simulink model "SingleTrack"  (R2019b)
settings: Solver=ode1  StartTime=0  StopTime=250  FixedStep=1.0000000000000000e-003  RelTol=1e-3
InitFcn:
  | sampleTime = str2double(get_param(bdroot, 'FixedStep'));
undefined symbols (not defined in the file or in its folder): AccPedalPos, BrakePedalPos, BrakeSwitch, DiscIntNeverNeededParam, DYNA4, EngSpd, IgnitionSwitch, InitialGear, InitialSpeed, IntendedEngTrq, LeftIndicator, MainBrakePress, MaxGear, MDL, MinGear, RefAcc, RefLane, RefLatPos, RefPath, RefPathCurv, RefSpd, RefSpdPreview, RefSpdRetrospect, RightIndicator, SteeringWheelAng, SteeringWheelTrq, UserDefinedRefValue, vm_const
libraries: UtilitiesLibrary x31, simulink x18, WheelSystemModules x13, LongitudinalControllerModules x13, LateralControllerModules x7, AnimationBusselectorModules x5, EnvironmentModules x5, BasicEngineControlModules x5, MiscellaneousControlModules x5, Animation3Modules x4, AuxiliariesModules x4, ReducedTireModules x4
(part 32 of 32)

== system SingleTrack/VehicleControl/LongitudinalControl/ControlSystems/Longitudinal Controller/Speed Control/Load Torque Vehicle ==
  VehSpd[m/s] : Inport
  TireRadius[m] : Inport  Port=2
  AerodynamicFrc[N] : Inport  Description=Vehicle Velocity  Port=3
  RoadSlopeLong [-] : Inport  Port=4
  SumMaxRollResistanceTrq[Nm] : Inport  Description=Vehicle Velocity  Port=5
  VehMass [kg] : Inport  Port=6
  BrakeFrc[N] : Inport  Port=7
  Constant : Constant  Value=9.81
  F_load [N] : Sum  Inputs=3  SaturateOnIntegerOverflow=on  InputSameDT=on  OutDataTypeStr=Inherit: Same as first input
  LoadTrq : Product  SaturateOnIntegerOverflow=on  InputSameDT=on  OutDataTypeStr=Inherit: Same as first input
  Resist.Torque : Product  SaturateOnIntegerOverflow=on  InputSameDT=on  OutDataTypeStr=Inherit: Same as first input
  Slope Force : Product  Inputs=3  SaturateOnIntegerOverflow=on  InputSameDT=on  OutDataTypeStr=Inherit: Same as first input
  Trigonometric Function : Trigonometry
  Trigonometric Function1 : Trigonometry  Operator=atan
  abs(F_load) [N]1 : Sum  Inputs=2  SaturateOnIntegerOverflow=on  InputSameDT=on  OutDataTypeStr=Inherit: Same as first input
  fade out load torque if speed is zero : Saturate  UpperLimit=1  LowerLimit=0
  toCompile : Subsystem  Tag=em_compile_service
      settings: AttributesFormatString=Place this block in the subsystem\n you want to compile
  LoadTrq[Nm] : Outport  VectorParamsAs1DForOutWhenUnconnected=off
  wires:
  VehSpd[m/s]/1 -> fade out load torque if speed is zero/1
  SumMaxRollResistanceTrq[Nm]/1 -> abs(F_load) [N]1/2
  TireRadius[m]/1 -> Resist.Torque/2
  Slope Force/1 -> F_load [N]/3
  Trigonometric Function/1 -> Slope Force/3
  VehMass [kg]/1 -> Slope Force/2
  Constant/1 -> Slope Force/1
  AerodynamicFrc[N]/1 -> F_load [N]/1
  BrakeFrc[N]/1 -> F_load [N]/2
  Resist.Torque/1 -> abs(F_load) [N]1/1
  RoadSlopeLong [-]/1 -> Trigonometric Function1/1
  F_load [N]/1 -> Resist.Torque/1
  abs(F_load) [N]1/1 -> LoadTrq/2
  fade out load torque if speed is zero/1 -> LoadTrq/1
  LoadTrq/1 -> LoadTrq[Nm]/1
  Trigonometric Function1/1 -> Trigonometric Function/1

== system SingleTrack/VehicleControl/LongitudinalControl/ControlSystems/Longitudinal Controller/Speed Control/Preprocessing VehicleInfo ==
  VehicleInfo : Inport
  Abs : Abs
  Add3 : Sum  Inputs=++++
  Add4 : Sum
  AverageRadius : Gain  Gain=0.25
  Bus Selector : BusSelector  OutputSignals=VehicleDriverInfo_TorqueRatio[-],VehicleDriverInfo_AccPedalPos[0_1],VehicleDriverInfo_OverallMass[kg],Chassis_VehicleBody_AbsVel[m/s],Drivetrain_DrivetrainPhysics_EngSpd[rad/s],Drivetrain_DrivetrainPhysics_Clutch_Pos[0_1],Drivetrain_DrivetrainPhysics_Transmission_Gear[-4;20],VehicleDriverInfo_TransmissionType[-],Auxiliaries_StarterTrq[Nm],VehicleDriverInfo_SumWheelRotAxisInrt[kg*m**2],Chassis_VehicleBody_AeroFrc(VehSys)[N],VehicleDriverInfo_SumMaxRollingResistanceTrq[Nm],VehicleDriverInfo_MaxDeceleration[m/s**2],WheelSystem_FrontLeft_Tire_DynamicRadius[m],WheelSystem_FrontRight_Tire_DynamicRadius[m],WheelSystem_RearLeft_Tire_DynamicRadius[m],WheelSystem_RearRight_Tire_DynamicRadius[m],VehicleDriverInfo_LongAeroDragCoeff[-],VehicleRoadInfo_RoadSlopeLong[-],VehicleDriverInfo_EngInrt[kg*m**2],VehicleDriverInfo_FullAccPedalTrq[Nm],VehicleDriverInfo_ZeroAccPedalTrq[Nm]
  DetectGearChange : Subsystem
  Product : Product  Inputs=***  RndMeth=Zero
  Product2 : Product  Inputs=**  RndMeth=Zero
  Saturation : Saturate  UpperLimit=1e6  LowerLimit=0.1
  Select x_value : Selector  InputPortWidth=3  IndexOptions=Index vector (dialog)  Indices=1  OutputSizes=1
  TractionCtrl : Subsystem
  factor from vehicle data : Gain  Gain=-1
  VehSpd[m/s] : Outport  VectorParamsAs1DForOutWhenUnconnected=off
  EngSpd[rad/s] : Outport  Port=2  VectorParamsAs1DForOutWhenUnconnected=off
  ExternalTrqs[Nm] : Outport  Port=3  VectorParamsAs1DForOutWhenUnconnected=off
  DynamicTireRadius[m] : Outport  Port=4  VectorParamsAs1DForOutWhenUnconnected=off
  VehAndWheelInrtl[kg*m**2] : Outport  Port=5  VectorParamsAs1DForOutWhenUnconnected=off
  TractionCtrlFlag[0/1] : Outport  Port=6  VectorParamsAs1DForOutWhenUnconnected=off
  MaxBrakeFrc[N] : Outport  Port=7  VectorParamsAs1DForOutWhenUnconnected=off
  FinalDriveRatio[-] : Outport  Port=8  VectorParamsAs1DForOutWhenUnconnected=off
  LongAeroDragCoeff[-] : Outport  Port=9  VectorParamsAs1DForOutWhenUnconnected=off
  AccPedalPos[0_1] : Outport  Port=10  VectorParamsAs1DForOutWhenUnconnected=off
  ClutchPos[0_1] : Outport  Port=11  VectorParamsAs1DForOutWhenUnconnected=off
  EngInrtl[kg*m**2] : Outport  Port=12  VectorParamsAs1DForOutWhenUnconnected=off
  Gear[-4;20] : Outport  Port=13  OutDataTypeStr=double  VectorParamsAs1DForOutWhenUnconnected=off
  FullAccPedalTrq[Nm] : Outport  Port=14  VectorParamsAs1DForOutWhenUnconnected=off
  ZeroAccPedalTrq[Nm] : Outport  Port=15  VectorParamsAs1DForOutWhenUnconnected=off
  AerodynamicFrc[N] : Outport  Port=16  VectorParamsAs1DForOutWhenUnconnected=off
  RoadSlopeLong[-] : Outport  Port=17  VectorParamsAs1DForOutWhenUnconnected=off
  SumMaxRollResistanceTrq[Nm] : Outport  Port=18  VectorParamsAs1DForOutWhenUnconnected=off
  VehMass[kg] : Outport  Port=19  VectorParamsAs1DForOutWhenUnconnected=off
  wires:
  Bus Selector/22 -> ZeroAccPedalTrq[Nm]/1  "<VehicleDriverInfo_ZeroAccPedalTrq[Nm]>"
  Bus Selector/21 -> FullAccPedalTrq[Nm]/1  "<VehicleDriverInfo_FullAccPedalTrq[Nm]>"
  Bus Selector/20 -> EngInrtl[kg*m**2]/1  "<VehicleDriverInfo_EngInrt[kg*m**2]>"
  VehicleInfo/1 -> Bus Selector/1
  Bus Selector/2 -> AccPedalPos[0_1]/1  "<VehicleDriverInfo_AccPedalPos[0_1]>"
  Bus Selector/7 -> Gear[-4;20]/1, DetectGearChange/1(Gear)  "<Drivetrain_DrivetrainPhysics_Transmission_Gear[-4;20]>"
  Bus Selector/8 -> DetectGearChange/2(TransmissionType)  "<VehicleDriverInfo_TransmissionType[-]>"
  Bus Selector/4 -> VehSpd[m/s]/1  "<Chassis_VehicleBody_AbsVel[m/s]>"
  Saturation/1 -> Product/3, Product/2, DynamicTireRadius[m]/1
  AverageRadius/1 -> Saturation/1
  TractionCtrl/1(ASRFlag [0/1]) -> TractionCtrlFlag[0/1]/1
  DetectGearChange/1(GearChangeFlag) -> TractionCtrl/2(GearChangeFlag [0|1])
  Product/1 -> Add4/1
  factor from vehicle data/1 -> AerodynamicFrc[N]/1
  Product2/1 -> MaxBrakeFrc[N]/1
  Add3/1 -> AverageRadius/1
  Add4/1 -> VehAndWheelInrtl[kg*m**2]/1
  Bus Selector/19 -> RoadSlopeLong[-]/1  "<VehicleRoadInfo_RoadSlopeLong[-]>"
  Abs/1 -> FinalDriveRatio[-]/1
  Bus Selector/1 -> Abs/1  "<VehicleDriverInfo_TorqueRatio[-]>"
  Bus Selector/3 -> Product/1, Product2/1, VehMass[kg]/1  "<VehicleDriverInfo_OverallMass[kg]>"
  Bus Selector/5 -> EngSpd[rad/s]/1  "<Drivetrain_DrivetrainPhysics_EngSpd[rad/s]>"
  Bus Selector/6 -> TractionCtrl/1(ClutchManual [0_1]), ClutchPos[0_1]/1  "<Drivetrain_DrivetrainPhysics_Clutch_Pos[0_1]>"
  Bus Selector/9 -> ExternalTrqs[Nm]/1  "<Auxiliaries_StarterTrq[Nm]>"
  Bus Selector/10 -> Add4/2  "<VehicleDriverInfo_SumWheelRotAxisInrt[kg*m**2]>"
  Bus Selector/11 -> Select x_value/1  "<Chassis_VehicleBody_AeroFrc(VehSys)[N]>"
  Select x_value/1 -> factor from vehicle data/1
  Bus Selector/12 -> SumMaxRollResistanceTrq[Nm]/1  "<VehicleDriverInfo_SumMaxRollingResistanceTrq[Nm]>"
  Bus Selector/13 -> Product2/2  "<VehicleDriverInfo_MaxDeceleration[m/s**2]>"
  Bus Selector/14 -> Add3/1  "<WheelSystem_FrontLeft_Tire_DynamicRadius[m]>"
  Bus Selector/15 -> Add3/2  "<WheelSystem_FrontRight_Tire_DynamicRadius[m]>"
  Bus Selector/16 -> Add3/3  "<WheelSystem_RearLeft_Tire_DynamicRadius[m]>"
  Bus Selector/17 -> Add3/4  "<WheelSystem_RearRight_Tire_DynamicRadius[m]>"
  Bus Selector/18 -> LongAeroDragCoeff[-]/1  "<VehicleDriverInfo_LongAeroDragCoeff[-]>"

== system SingleTrack/VehicleControl/LongitudinalControl/ControlSystems/Longitudinal Controller/Speed Control/Write to ControlOutputs ==
  AccPedalPos[0_1] : Inport
  IntendedEngTrq[Nm] : Inport  Port=2
  EngSpd[rad/s] : Inport  Port=3
  RefSpd[m/s] : Inport  Port=4
  RefAcc[m/s**2] : Inport  Port=5
  BrakePedalPos[0_1] : Inport  Port=6
  Bus Assignment : BusAssignment  AssignedSignals=AccPedalPos,BrakePedalPos,IntendedEngTrq,EngSpd,RefSpd,RefAcc
  Create SpeedControlOutput Bus : Constant  Value=0  OutDataTypeStr=Bus: TD_BO_LongitudinalSpeedControlOutputs
  ControlOutputs : Outport  VectorParamsAs1DForOutWhenUnconnected=off
  wires:
  RefSpd[m/s]/1 -> Bus Assignment/6  "RefSpd[m/s]"
  EngSpd[rad/s]/1 -> Bus Assignment/5  "EngSpd[rad/s]"
  IntendedEngTrq[Nm]/1 -> Bus Assignment/4  "IntendedEngTrq[Nm]"
  BrakePedalPos[0_1]/1 -> Bus Assignment/3  "BrakePedalPos[0_1]"
  AccPedalPos[0_1]/1 -> Bus Assignment/2  "AccPedalPos[0_1]"
  Bus Assignment/1 -> ControlOutputs/1
  Create SpeedControlOutput Bus/1 -> Bus Assignment/1
  RefAcc[m/s**2]/1 -> Bus Assignment/7  "RefAcc[m/s**2]"

== system SingleTrack/VehicleControl/LongitudinalControl/ControlSystemsPreprocessor/Generation of Speed Data/Smooth Derivative/Transfer Fcn with variable prameter ==
  note: Transfer function with variable parameters:
      | num = s
      | den = T^2*s^2 + 2*T*s + 1
      |
      | H(s) = Y(s) / U(s) = s / (T^2*s^2 + 2*T*s + 1)
      | -->
      | Y(s) = 1/T^2*1/s*U(s) - 2/T*1/s*Y(s) - 1/T^2*1/s^2*Y(s)
  u : Inport
  T : Inport  Port=2
  Add : Sum  Inputs=+--
  Discrete-Time Integrator : DiscreteIntegrator  InitialConditionSource=external  SampleTime=-1  ICPrevOutput=DiscIntNeverNeededParam  ICPrevScaledInput=DiscIntNeverNeededParam
  Discrete-Time Integrator1 : DiscreteIntegrator  InitialConditionSource=external  SampleTime=-1  ICPrevOutput=DiscIntNeverNeededParam  ICPrevScaledInput=DiscIntNeverNeededParam
  Discrete-Time Integrator2 : DiscreteIntegrator  SampleTime=-1  ICPrevOutput=DiscIntNeverNeededParam  ICPrevScaledInput=DiscIntNeverNeededParam
  Gain : Gain  Gain=2
  Gain2 : Gain  Gain=2
  Product1 : Product  Inputs=3
  Product2 : Product  Inputs=3
  Product3 : Product
  Product4 : Product
  Reciprocal : Product  Inputs=/
  y : Outport  VectorParamsAs1DForOutWhenUnconnected=off
  wires:
  Add/1 -> y/1, Discrete-Time Integrator1/1
  Product3/1 -> Gain/1
  T/1 -> Product4/2, Reciprocal/1
  Gain/1 -> Add/3
  Reciprocal/1 -> Product1/3, Product1/2, Product2/3, Product3/2, Product2/2
  Product2/1 -> Add/2
  Product1/1 -> Add/1
  Discrete-Time Integrator/1 -> Product1/1
  Discrete-Time Integrator2/1 -> Product2/1
  Discrete-Time Integrator1/1 -> Discrete-Time Integrator2/1, Product3/1
  Product4/1 -> Gain2/1
  u/1 -> Discrete-Time Integrator/1, Discrete-Time Integrator1/2, Product4/1
  Gain2/1 -> Discrete-Time Integrator/2

== system SingleTrack/VehicleControl/LateralControl/Disabled LateralControl/ControlSystems/Control Systems Parameters/CurvatureControl/DynaModuleInfo ==

== system SingleTrack/VehicleControl/LateralControl/Disabled LateralControl/ControlSystems/Control Systems Parameters/PathControl/DynaModuleInfo ==

== system SingleTrack/VehicleControl/LateralControl/Disabled LateralControl/ControlSystems/Lateral Controller/User-Defined Control/UserDefinedControl ==
  DynaModuleInfo : Subsystem  Tag=DynaModuleInfo
      mask init:
      | data = get_param(gcb, 'UserData');
      mask Display:
      | disp(['Type = ', data.type, '\nName = ', char(data.name)
      | ]);

== system SingleTrack/VehicleControl/LongitudinalControl/ControlSystems/Longitudinal Controller/Acceleration Control/ComputeBrakePedalPos/Calculate Brake Pedal ==
  Factor_TyreTorque_2_BrakePedalPosition : Inport
  Int Torque on Wheel : Inport  Port=2
  Constant1 : Constant  Value=0
  Divide : Product  Inputs=*/
  Gain : Gain  Gain=-1
  Limiter [0-1] : Subsystem
  Relational Operator : RelationalOperator  Operator=<  OutDataTypeStr=boolean  RndMeth=Nearest
  Switch : Switch  Threshold=0.5
  Brake Pedal Position : Outport  VectorParamsAs1DForOutWhenUnconnected=off
  wires:
  Limiter [0-1]/1(Out) -> Brake Pedal Position/1
  Int Torque on Wheel/1 -> Relational Operator/1, Gain/1
  Divide/1 -> Limiter [0-1]/1(In)
  Switch/1 -> Divide/1
  Gain/1 -> Switch/1
  Relational Operator/1 -> Switch/2
  Constant1/1 -> Switch/3, Relational Operator/2
  Factor_TyreTorque_2_BrakePedalPosition/1 -> Divide/2

== system SingleTrack/VehicleControl/LongitudinalControl/ControlSystems/Longitudinal Controller/Acceleration Control/ComputeBrakePedalPos/Factor_TyreTorque_2_BrakePedalPosition ==
  VehicleInfo : Inport
  Bus Selector3 : BusSelector  OutputSignals=VehicleDriverInfo_MaxMainBrakePress[Pa],WheelSystem_FrontLeft_Wheel_BrakeTrqPressRatio[m**3],WheelSystem_FrontRight_Wheel_BrakeTrqPressRatio[m**3],WheelSystem_RearLeft_Wheel_BrakeTrqPressRatio[m**3],WheelSystem_RearRight_Wheel_BrakeTrqPressRatio[m**3]
  Divide : Product  Inputs=**
  Sum of Elements : Sum  Inputs=++++
  Factor_TyreTorque_2_BrakePedalPosition : Outport  VectorParamsAs1DForOutWhenUnconnected=off
  wires:
  VehicleInfo/1 -> Bus Selector3/1
  Bus Selector3/1 -> Divide/1  "<VehicleDriverInfo_MaxMainBrakePress[Pa]>"
  Divide/1 -> Factor_TyreTorque_2_BrakePedalPosition/1
  Bus Selector3/2 -> Sum of Elements/1  "<WheelSystem_FrontLeft_Wheel_BrakeTrqPressRatio[m**3]>"
  Bus Selector3/3 -> Sum of Elements/2  "<WheelSystem_FrontRight_Wheel_BrakeTrqPressRatio[m**3]>"
  Bus Selector3/4 -> Sum of Elements/3  "<WheelSystem_RearLeft_Wheel_BrakeTrqPressRatio[m**3]>"
  Bus Selector3/5 -> Sum of Elements/4  "<WheelSystem_RearRight_Wheel_BrakeTrqPressRatio[m**3]>"
  Sum of Elements/1 -> Divide/2

== system SingleTrack/VehicleControl/LongitudinalControl/ControlSystems/Longitudinal Controller/Acceleration Control/ComputeBrakePedalPos/no Brake AND Gas ==
  AccPedal : Inport
  BrakePedal : Inport  Port=2
  PedalChangeTime : Inport  Port=3
  Constant3 : Constant  Value=1e-3
  Constant4 : Constant  Value=0
  Data Type Conversion : DataTypeConversion  OutDataTypeStr=double  SaturateOnIntegerOverflow=on  RndMeth=Zero
  Integrator : DiscreteIntegrator  ExternalReset=either  SampleTime=-1  ICPrevOutput=DiscIntNeverNeededParam  ICPrevScaledInput=DiscIntNeverNeededParam
  "Pedal Change Time " : RelationalOperator  RndMeth=Nearest  InputSameDT=on
      settings: AttributesFormatString===> Brake allowed
  Switch : Switch  Threshold=0.5
  no Gas1 : RelationalOperator  Operator=>  RndMeth=Nearest  InputSameDT=on
  ModifiedBrakePedalPos [0-1] : Outport  VectorParamsAs1DForOutWhenUnconnected=off
  wires:
  PedalChangeTime/1 -> "Pedal Change Time "/2
  Constant4/1 -> Switch/3
  BrakePedal/1 -> Switch/1
  Switch/1 -> ModifiedBrakePedalPos [0-1]/1
  Constant3/1 -> no Gas1/1
  Integrator/1 -> "Pedal Change Time "/1
  no Gas1/1 -> Data Type Conversion/1
  AccPedal/1 -> no Gas1/2
  "Pedal Change Time "/1 -> Switch/2
  Data Type Conversion/1 -> Integrator/2, Integrator/1

== system SingleTrack/VehicleControl/LongitudinalControl/ControlSystems/Longitudinal Controller/Speed Control/Load Torque Vehicle/toCompile ==

== system SingleTrack/VehicleControl/LongitudinalControl/ControlSystems/Longitudinal Controller/Speed Control/Preprocessing VehicleInfo/DetectGearChange ==
  note: TransmissionType
      | 0 = none
      | 1 = manual
      | 2 = automatic
  Gear : Inport
  TransmissionType : Inport  Port=2
  Data Type Conversion2 : DataTypeConversion  OutDataTypeStr=double
  Default : Constant  Value=0
  Multiport Switch : MultiPortSwitch  DataPortOrder=Zero-based contiguous  Inputs=4  zeroidx=on
  if gear change : RelationalOperator  Operator=~=  OutDataTypeStr=boolean  RndMeth=Nearest  InputSameDT=on
  if neither selected nor previous gear zero : Logic  AllPortsSameDT=off  OutDataTypeStr=boolean
  if neither selected nor previous gear zero1 : Logic
  previous gear : Memory  InheritSampleTime=on
  GearChangeFlag : Outport  VectorParamsAs1DForOutWhenUnconnected=off
  wires:
  if neither selected nor previous gear zero/1 -> if neither selected nor previous gear zero1/2
  if gear change/1 -> if neither selected nor previous gear zero1/1
  Data Type Conversion2/1 -> GearChangeFlag/1
  Gear/1 -> Multiport Switch/5, Multiport Switch/3, Multiport Switch/4  "selected gear"
  Default/1 -> Multiport Switch/2
  TransmissionType/1 -> Multiport Switch/1
  if neither selected nor previous gear zero1/1 -> Data Type Conversion2/1  "gear change (not from/to neutral)"
  Multiport Switch/1 -> previous gear/1, if neither selected nor previous gear zero/2, if gear change/1  "selected gear"
  previous gear/1 -> if neither selected nor previous gear zero/1, if gear change/2  "previous gear"

== system SingleTrack/VehicleControl/LongitudinalControl/ControlSystems/Longitudinal Controller/Speed Control/Preprocessing VehicleInfo/TractionCtrl ==
  ClutchManual [0_1] : Inport
  GearChangeFlag [0|1] : Inport  Port=2
  Constant : Constant  Value=1e-5
  Data Type Conversion : DataTypeConversion  OutDataTypeStr=double  SaturateOnIntegerOverflow=on  RndMeth=Zero
  Data Type Conversion1 : DataTypeConversion  OutDataTypeStr=boolean  SaturateOnIntegerOverflow=on  RndMeth=Zero
  Data Type Conversion2 : DataTypeConversion  OutDataTypeStr=boolean  SaturateOnIntegerOverflow=on  RndMeth=Zero
  Data Type Conversion3 : DataTypeConversion  OutDataTypeStr=double  SaturateOnIntegerOverflow=on  RndMeth=Zero
  Hit Crossing : HitCross  HitCrossingOffset=0.5  HitCrossingDirection=rising
  Relational Operator : RelationalOperator  Operator=>  RndMeth=Nearest
  S-R Flip-Flop : simulink_extras/Flip Flops/S-R Flip-Flop  initial_condition=0
  Terminator : Terminator
  ASRFlag [0/1] : Outport  VectorParamsAs1DForOutWhenUnconnected=off
  wires:
  GearChangeFlag [0|1]/1 -> Data Type Conversion1/1
  S-R Flip-Flop/1 -> Data Type Conversion/1
  Data Type Conversion/1 -> ASRFlag [0/1]/1
  S-R Flip-Flop/2 -> Terminator/1
  ClutchManual [0_1]/1 -> Relational Operator/1
  Constant/1 -> Relational Operator/2
  Relational Operator/1 -> Data Type Conversion3/1
  Hit Crossing/1 -> Data Type Conversion2/1
  Data Type Conversion1/1 -> S-R Flip-Flop/1
  Data Type Conversion2/1 -> S-R Flip-Flop/2
  Data Type Conversion3/1 -> Hit Crossing/1

== system SingleTrack/VehicleControl/LateralControl/Disabled LateralControl/ControlSystems/Lateral Controller/User-Defined Control/UserDefinedControl/DynaModuleInfo ==

== system SingleTrack/VehicleControl/LongitudinalControl/ControlSystems/Longitudinal Controller/Acceleration Control/ComputeBrakePedalPos/Calculate Brake Pedal/Limiter [0-1] ==
  In : Inport
  Limiter : MinMax  Inputs=2  SaturateOnIntegerOverflow=on  InputSameDT=on
  Limiter1 : MinMax  Function=max  Inputs=2  SaturateOnIntegerOverflow=on  InputSameDT=on
  max. brake pedal position : Constant
  min. brake pedal position : Constant  Value=0
  Out : Outport  VectorParamsAs1DForOutWhenUnconnected=off
  wires:
  max. brake pedal position/1 -> Limiter/2
  Limiter/1 -> Limiter1/1
  min. brake pedal position/1 -> Limiter1/2
  In/1 -> Limiter/1
  Limiter1/1 -> Out/1
